simulink model "self_balance_alone"  (R2023b)
settings: Solver=VariableStepAuto  StartTime=0.0  StopTime=10.0  RelTol=1e-3
undefined symbols (not defined in the file): den, num, thetaddot_add, thetaddot_coeff, thetaddot_theta_coeff, thetaddot_xdot_coeff, xddot_coeff, xddot_theta_coeff, xddot_xdot_coeff
settings Model: Creator=emamaker  LastModifiedBy=emamaker

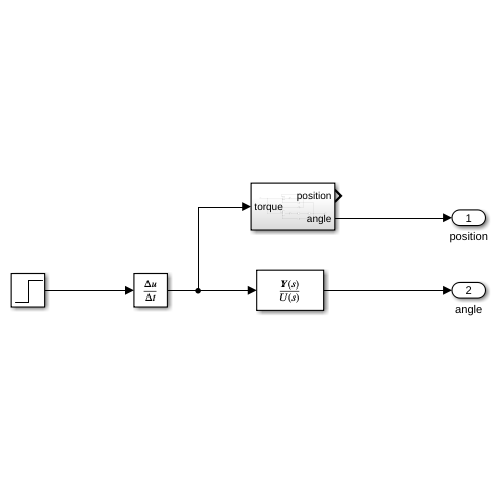
[thumbnail: Simulink's stored preview of the top-level diagram]
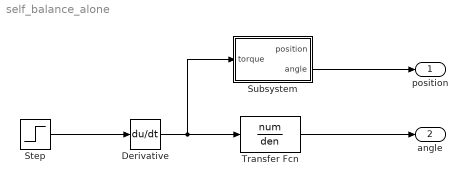
== system self_balance_alone ==
  Derivative : Derivative
  Step : Step  After=0.1  SampleTime=0
  Subsystem : Subsystem
  Transfer Fcn : TransferFcn  Numerator=num  Denominator=den
  position : Outport
  angle : Outport  Port=2
  wires:
  Step/1 -> Derivative/1
  Derivative/1 -> Subsystem/1(torque), Transfer Fcn/1
  Transfer Fcn/1 -> angle/1
  Subsystem/2(angle) -> position/1

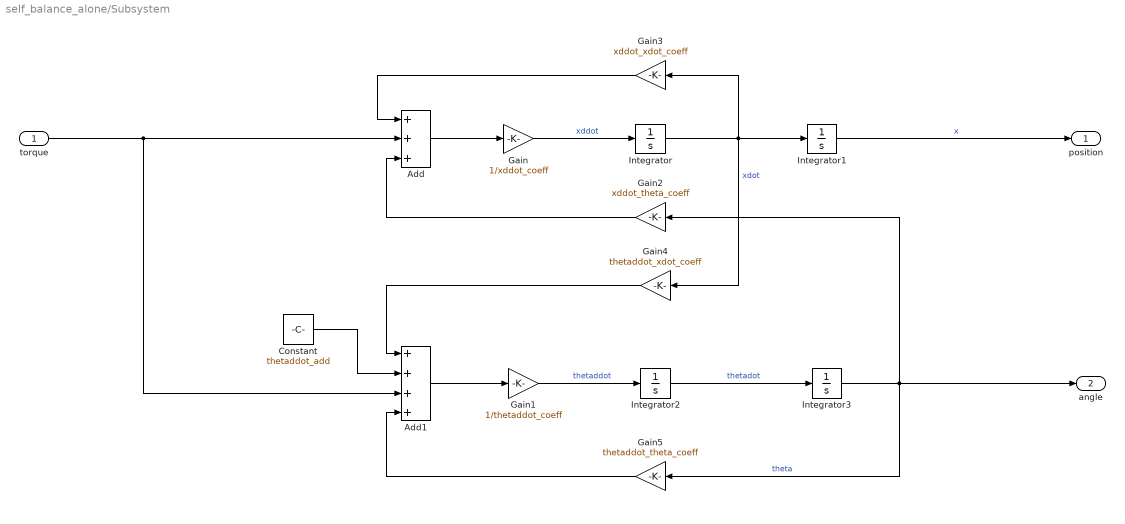
== system self_balance_alone/Subsystem ==
  torque : Inport
  Add : Sum  Inputs=+++
  Add1 : Sum  Inputs=++++
  Constant : Constant  Value=thetaddot_add
  Gain : Gain  Gain=1/xddot_coeff
  Gain1 : Gain  Gain=1/thetaddot_coeff
  Gain2 : Gain  Gain=xddot_theta_coeff
  Gain3 : Gain  Gain=xddot_xdot_coeff
  Gain4 : Gain  Gain=thetaddot_xdot_coeff
  Gain5 : Gain  Gain=thetaddot_theta_coeff
  Integrator{,1..3} (4 alike) : Integrator
  position : Outport
  angle : Outport  Port=2
  wires:
  Integrator1/1 -> position/1  "x"
  Gain1/1 -> Integrator2/1  "thetaddot"
  Integrator3/1 -> angle/1, Gain5/1, Gain2/1  "theta"
  Gain4/1 -> Add1/1
  Gain/1 -> Integrator/1  "xddot"
  Add1/1 -> Gain1/1
  torque/1 -> Add1/3, Add/2
  Integrator/1 -> Gain4/1, Gain3/1, Integrator1/1  "xdot"
  Integrator2/1 -> Integrator3/1  "thetadot"
  Gain3/1 -> Add/1
  Gain2/1 -> Add/3
  Add/1 -> Gain/1
  Gain5/1 -> Add1/4
  Constant/1 -> Add1/2
